simulink model "sldemo_varsize_basic"  (Simulink 7.6)
settings: Solver=FixedStepDiscrete  StartTime=0.0  StopTime=10.0  RelTol=1e-3
undefined symbols (not defined in the file or in its folder): j
libraries: simulink x1
settings Model: Creator=The MathWorks Inc.
settings DataIOCC: SaveFormat=Structure  SaveState=on

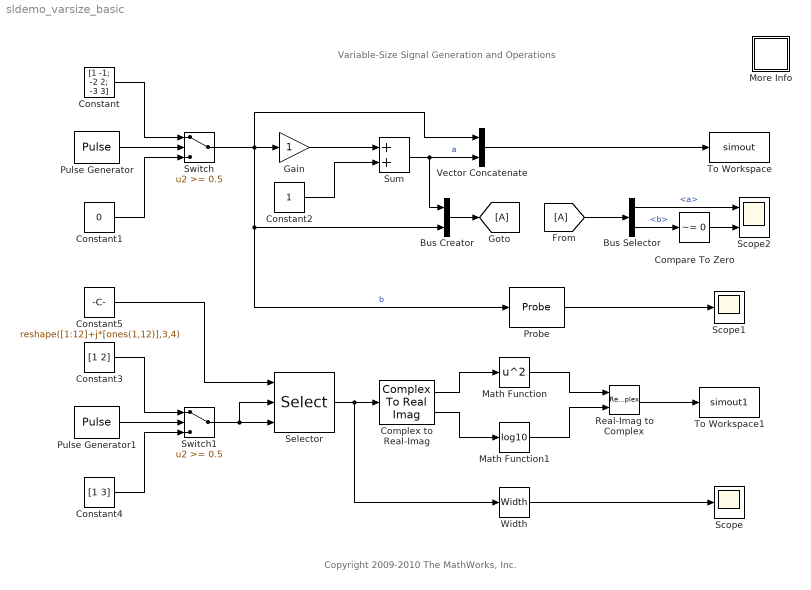
== system sldemo_varsize_basic ==
  note: Variable-Size Signal Generation and Operations
  note: Copyright 2009-2010 The MathWorks, Inc.
  Bus Creator : BusCreator  Inputs=2
  Bus Selector : BusSelector  OutputSignals=a,b
  Compare To Zero : simulink/Logic and Bit Operations/Compare To Zero  SystemSampleTime=-1  relop=~=  LogicOutDataTypeMode=uint8
  Complex to Real-Imag : ComplexToRealImag
  Constant : Constant  Value=[1 -1; -2 2; -3 3]
  Constant1 : Constant  Value=0
  Constant2 : Constant
  Constant3 : Constant  Value=[1 2]
  Constant4 : Constant  Value=[1 3]
  Constant5 : Constant  Value=reshape([1:12]+j*[ones(1,12)],3,4)
  Gain : Gain
  Math Function : Math  Operator=square  SaturateOnIntegerOverflow=on
  Math Function1 : Math  Operator=log10  SaturateOnIntegerOverflow=on
  More Info : Subsystem
      settings: OpenFcn=showdemo(bdroot(gcb))
      mask Display: disp('?')
  Probe : Probe  ProbeWidth=off  ProbeSampleTime=off  ProbeComplexSignal=off  ProbeSignalDimensions=on
  Pulse Generator : DiscretePulseGenerator  Period=4  PulseWidth=2
  Pulse Generator1 : DiscretePulseGenerator  Period=4  PulseWidth=2
  Real-Imag to Complex : RealImagToComplex
  Scope : Scope
      settings: YMin=3  YMax=10
  Scope1 : Scope
      settings: YMin=0  YMax=4
  Scope2 : Scope  NumInputPorts=2
      settings: TimeRange=10  YMin=-3~-0.5  YMax=5~1.5  SaveName=ScopeData2
  Selector : Selector  NumberOfDimensions=2  InputPortWidth=3  IndexOptions=Starting and ending indices (port),Starting and ending indices (port)  Indices=[1 3],1  OutputSizes=1,1
  Sum : Sum
  Switch : Switch  Threshold=0.5  AllowDiffInputSizes=on
  Switch1 : Switch  Threshold=0.5
  To Workspace : ToWorkspace  VariableName=simout  SampleTime=-1  SaveFormat=Structure
  To Workspace1 : ToWorkspace  VariableName=simout1  SampleTime=-1  SaveFormat=Structure
  Vector Concatenate : Concatenate  Mode=Multidimensional array
  Width : Width
  wires:
  Constant/1 -> Switch/1
  Pulse Generator/1 -> Switch/2
  Constant1/1 -> Switch/3
  Switch/1 -> Gain/1, Vector Concatenate/1, Probe/1, Bus Creator/2  "b"
  Constant3/1 -> Switch1/1
  Pulse Generator1/1 -> Switch1/2
  Constant4/1 -> Switch1/3
  Switch1/1 -> Selector/3, Selector/2
  Constant5/1 -> Selector/1
  Selector/1 -> Width/1, Complex to Real-Imag/1
  Real-Imag to Complex/1 -> To Workspace1/1
  Width/1 -> Scope/1
  Math Function1/1 -> Real-Imag to Complex/2
  Complex to Real-Imag/2 -> Math Function1/1
  Math Function/1 -> Real-Imag to Complex/1
  Complex to Real-Imag/1 -> Math Function/1
  Sum/1 -> Vector Concatenate/2, Bus Creator/1  "a"
  Vector Concatenate/1 -> To Workspace/1
  Constant2/1 -> Sum/2
  Gain/1 -> Sum/1
  Probe/1 -> Scope1/1
  Compare To Zero/1 -> Scope2/2
  Bus Selector/2 -> Compare To Zero/1  "<b>"
  Bus Selector/1 -> Scope2/1  "<a>"
  Bus Creator/1 -> [A]
  [A] -> Bus Selector/1

== system sldemo_varsize_basic/More Info ==
  note: This demonstration shows how signals may be grouped and ungrouped while
      | retaining their names.  In this demonstration, 5 signals are created and labelled
      | appropriately.  These signals are then mux'd together to create a bus of signals.
      | This bus of signals is then fed into the Bus Selector block.  Inside of the Bus
      | Selector block, the Pulse and Chirp signals are chosen to be output from the
      | original signal bus.
      |
      | It is possible to place a nest signal buses and then still retrieve the original signal
      | with its label.
  note: Bus Block Demonstration
